simulink model "cube_3d_simulation_model"  (R2016a)
settings: Solver=VariableStepAuto  StartTime=0.0  StopTime=10.0  MaxStep=0.0001  RelTol=1e-3
values from neighbouring files (symbols this model uses):
  Q0 = Q0/norm(Q0)    [run_simulation_3D.m]
settings Model: Creator=Love  LastModifiedBy=Love

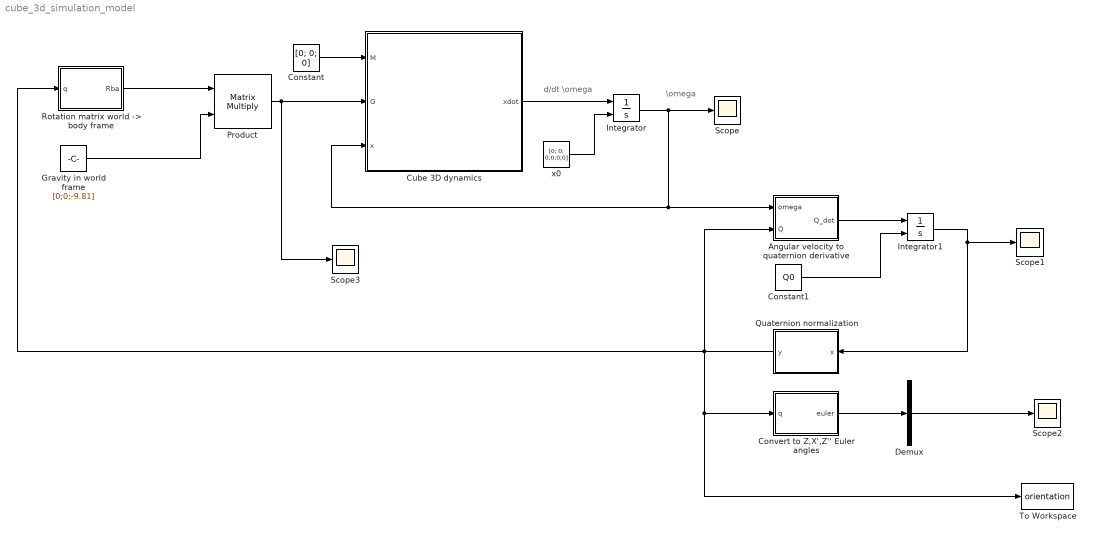
== system cube_3d_simulation_model ==
  note: \omega
  note: d/dt \omega
  Angular velocity to quaternion derivative : MATLAB Function  TreatAsAtomicUnit=on
  Constant : Constant  Value=[0; 0; 0]
  Constant1 : Constant  Value=Q0
  Convert to Z,X',Z'' Euler angles : MATLAB Function  TreatAsAtomicUnit=on
  Cube 3D dynamics : MATLAB Function  TreatAsAtomicUnit=on
  Demux : Demux  Outputs=3
  Gravity in world frame : Constant  Value=[0;0;-9.81]
  Integrator : Integrator  InitialConditionSource=external
  Integrator1 : Integrator  InitialConditionSource=external
  Product : Product  Multiplication=Matrix(*)
  Quaternion normalization : MATLAB Function  TreatAsAtomicUnit=on
  "Rotation matrix world -> body frame" : MATLAB Function  TreatAsAtomicUnit=on
  Scope{,1..3} (4 alike) : Scope
  To Workspace : ToWorkspace  VariableName=orientation  SaveFormat=Timeseries  SampleTime=-1
  x0 : Constant  Value=[0; 0; 0;0;0;0]
  wires:
  Cube 3D dynamics/1(xdot) -> Integrator/1
  Integrator/1 -> Scope/1, Cube 3D dynamics/3(x), Angular velocity to quaternion derivative/1(omega)
  Constant/1 -> Cube 3D dynamics/1(M)
  x0/1 -> Integrator/2
  Angular velocity to quaternion derivative/1(Q_dot) -> Integrator1/1
  Constant1/1 -> Integrator1/2
  Integrator1/1 -> Scope1/1, Quaternion normalization/1(x)
  Product/1 -> Scope3/1, Cube 3D dynamics/2(G)
  "Rotation matrix world -> body frame"/1(Rba) -> Product/1
  Gravity in world frame/1 -> Product/2
  Quaternion normalization/1(y) -> To Workspace/1, Convert to Z,X',Z'' Euler angles/1(q), "Rotation matrix world -> body frame"/1(q), Angular velocity to quaternion derivative/2(Q)
  Convert to Z,X',Z'' Euler angles/1(euler) -> Demux/1
  Demux/2 -> Scope2/1

== matlab function cube_3d_simulation_model/Angular velocity to quaternion derivative ==
  data: omega input; Q_dot output; Q input
function Q_dot = fcn(omega, Q)
%#codegen
    
   omega = omega(1:3); 
   q0=Q(1);   q1=Q(2);   q2=Q(3);   q3=Q(4);
   
   %The matrix that relates angular velocity in the body frame to the
   %quaternion derivatives. From : https://www.control.isy.liu.se/student/tsrt14/file/orientation.pdf 
   Sbar=[-q1    -q2     -q3;
          q0    -q3      q2;
          q3    q0      -q1;
         -q2    q1       q0];
    
    Q_dot = (0.5*Sbar*omega)';

== matlab function cube_3d_simulation_model/Cube 3D dynamics ==
  data: M input; G input; xdot output; x input; cube parameter
function xdot = fcn(M, G,x, cube)
%#codegen

w = x(1:3); 

%Eulers laws of rotation 
wdot = inv(cube.I3D)*(M + cross(cube.rcb,G) - cross(w, cross(w,cube.tensor*w))  );

xdot = [wdot ; 0; 0;0];

== matlab function cube_3d_simulation_model/Quaternion normalization ==
  data: x input; y output
function y = fcn(x)
%#codegen

%Reportedly, numerical errors can make quaternion loose their unit length
%property. This is the remedy.  

  x(1:4)  = x(1:4) / norm(x(1:4));
  
  %Enforce q0 -> 0 to avoid ambiguity 
  if x(1) < 0,
    x(1:4) = -x(1:4);
  end

y = x;

== matlab function cube_3d_simulation_model/Rotation matrix world -> body frame ==
  data: q input; Rba output
function Rba = fcn(q)
%#codegen

    R = zeros(3,3); %Added 3 dimensional result array for codegen
    
    R(1,1) = 2.*q(1).^2-1+2.*q(2).^2;
    R(1,2) = 2.*(q(2).*q(3)+q(1).*q(4));
    R(1,3) = 2.*(q(2).*q(4)-q(1).*q(3));
    R(2,1) = 2.*(q(2).*q(3)-q(1).*q(4));
    R(2,2) = 2.*q(1).^2-1+2.*q(3).^2;
    R(2,3) = 2.*(q(3).*q(4)+q(1).*q(2));
    R(3,1) = 2.*(q(2).*q(4)+q(1).*q(3));
    R(3,2) = 2.*(q(3).*q(4)-q(1).*q(2));
    R(3,3) = 2.*q(1).^2-1+2.*q(4).^2;

Rba = R';

== matlab function cube_3d_simulation_model/Convert to Z,X',Z'' Euler angles ==
  data: q input; euler output
function euler = fcn(q)
%#codegen

%Convert quaternions first to parts of rotation matrix and then to Z-X'-Z''
%euler angles. Note that the angles are not the same as used in for
%instance magdwick as standard! 


    R = zeros(3,3); %Added 3 dimensional result array for codegen  
    
    R(1,3) = 2.*(q(2).*q(4)-q(1).*q(3));
     R(2,3) = 2.*(q(3).*q(4)+q(1).*q(2));
    
    R(3,1) = 2.*(q(2).*q(4)+q(1).*q(3));
    R(3,2) = 2.*(q(3).*q(4)-q(1).*q(2));
    
    R(3,3) = 2.*q(1).^2-1+2.*q(4).^2;
    
    phi = atan2(R(1,3), R(2,3)); 
    theta = acos(R(3,3)); 
    psi = atan2(  R(3,1),R(3,2) );
    
    euler = [phi;theta;psi];
